simulink model "real_time_simulink_LQR"  (R2024b)
settings: Solver=ode5  StartTime=0.0  StopTime=4.5  FixedStep=0.001  RelTol=1e-3
values from neighbouring files (symbols this model uses):
  deltafil = 2^(-0.5)    (= 0.707106781187)    [LQR_code.m]    (also in PID_Luca.m)
  Klqr2 = lqr(sysG,Q,R)    [LQR_code.m]
  Nu = N(5)    [LQR_code.m]
  Nx = [N(1);N(2);N(3);N(4)]    [LQR_code.m]
  omegac = 2*pi*50    (= 314.159265359)    [LQR_code.m]    (also in PID_Luca.m)
  t0 = 0.2    [Elastic_parameters_estimation.m]    (also in LQR_code.m; PID_Luca.m)
  t1 = 0.7    [Elastic_parameters_estimation.m]    (also in LQR_code.m; PID_Luca.m)
undefined symbols (not defined in the file or in its folder): degs2rpm, DiscIntNeverNeededParam, National_Instruments, PCI, pulse2deg, rpm2rads
libraries: sldrtlib x3, simulink x3
settings Model: SimulationMode=external  ExtModeTrigDuration=1000001  Creator=galeazzolu  LastModifiedBy=galeazzolu
settings DataIOCC: ReturnWorkspaceOutputs=off
settings HardwareCC: ProdBitPerLong=64  ProdHWDeviceType=Intel->x86-64 (Linux 64)
settings RTWCC: Description=Simulink Desktop Real-Time  SystemTargetFile=sldrt.tlc  TemplateMakefile=sldrt.tmf  RTWCompilerOptimization=on
settings CodeAppCC: MaxIdLength=95
settings SimulinkDesktopRealTimeCC: TargetLibSuffix=_sldrt.a  TargetPreCompLibLocation=C:\Program Files\MATLAB\R2024b\toolbox\sldrt\lib\win64  ParMdlRefBuildCompliant=on

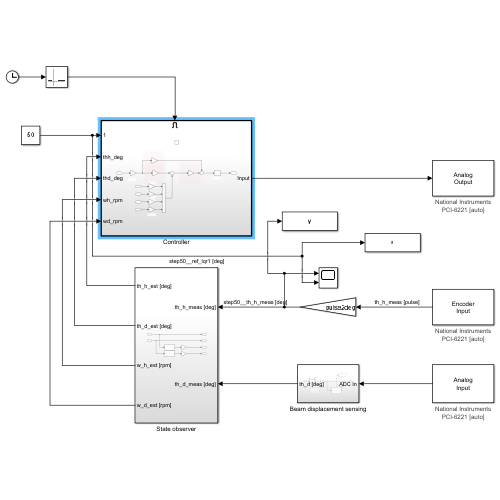
[thumbnail: Simulink's stored preview of the top-level diagram]
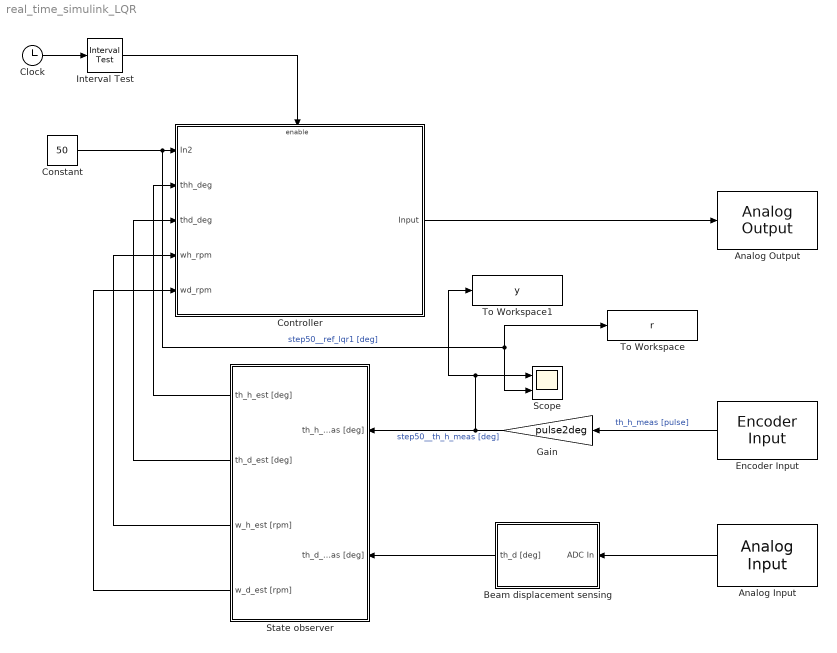
== system real_time_simulink_LQR ==
  Analog Input : sldrtlib/Analog Input  SampleTime=-1  MaxMissedTicks=10  ShowMissedTicks=off  YieldWhenWaiting=off  DrvName=National_Instruments/PCI-6221  DrvAddress=4294967295  DrvOptions=[0 0 0 2 0]  Channels=[3,4]  RangeMode=1  VoltRange=2  DataType=1
      settings: AttributesFormatString=National Instruments\nPCI-6221 [auto]
  Analog Output : sldrtlib/Analog Output  SampleTime=-1  MaxMissedTicks=10  ShowMissedTicks=off  YieldWhenWaiting=off  DrvName=National_Instruments/PCI-6221  DrvAddress=4294967295  DrvOptions=[0 0 0 2 0]  Channels=1  RangeMode=1  VoltRange=1  InitialValue=0  FinalValue=0
      settings: AttributesFormatString=National Instruments\nPCI-6221 [auto]
  Beam displacement sensing : Subsystem
  Clock : Clock
  Constant : Constant  Value=50
  Controller : Subsystem
  Encoder Input : sldrtlib/Encoder Input  SampleTime=-1  MaxMissedTicks=10  ShowMissedTicks=off  YieldWhenWaiting=off  DrvName=National_Instruments/PCI-6221  DrvAddress=4294967295  DrvOptions=[0 0 0 2 0]  Channels=1  QuadMode=3  IndexPulse=1  InputFilter=Inf  DataType=1
      settings: AttributesFormatString=National Instruments\nPCI-6221 [auto]
  Gain : Gain  Gain=pulse2deg
  Interval Test : simulink/Logic and Bit Operations/Interval Test  IntervalClosedRight=on  uplimit=inf  IntervalClosedLeft=on  lowlimit=0.7  OutDataTypeStr=boolean
  Scope : Scope  NumInputPorts=2
  State observer : Subsystem
  To Workspace : ToWorkspace  VariableName=r  SaveFormat=Structure With Time  SampleTime=-1
  To Workspace1 : ToWorkspace  VariableName=y  SaveFormat=Structure With Time  SampleTime=-1
  wires:
  Beam displacement sensing/1(th_d [deg]) -> State observer/2(th_d_meas [deg])
  Gain/1 -> To Workspace1/1, Scope/1, State observer/1(th_h_meas [deg])  "step50__th_h_meas [deg]"
  State observer/2(th_d_est [deg]) -> Controller/3(thd_deg)
  State observer/1(th_h_est [deg]) -> Controller/2(thh_deg)
  Encoder Input/1 -> Gain/1  "th_h_meas [pulse]"
  State observer/4(w_d_est [rpm]) -> Controller/5(wd_rpm)
  Analog Input/1 -> Beam displacement sensing/1(ADC In)
  State observer/3(w_h_est [rpm]) -> Controller/4(wh_rpm)
  Clock/1 -> Interval Test/1
  Interval Test/1 -> Controller/Enable
  Constant/1 -> To Workspace/1, Scope/2, Controller/1(In2)  "step50__ref_lqr1 [deg]"
  Controller/1(Input) -> Analog Output/1

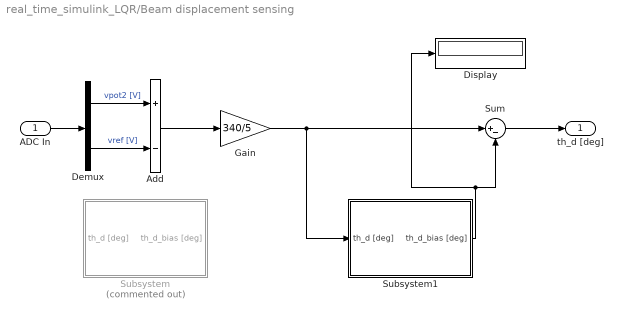
== system real_time_simulink_LQR/Beam displacement sensing ==
  ADC In : Inport
  Add : Sum  Inputs=+-
  Demux : Demux  Outputs=2
  Display : Display
  Gain : Gain  Gain=340/5
  Subsystem : Subsystem  Commented=on
  Subsystem1 : Subsystem
  Sum : Sum  Inputs=|+-
  th_d [deg] : Outport
  wires:
  ADC In/1 -> Demux/1
  Demux/1 -> Add/1  "vpot2 [V]"
  Demux/2 -> Add/2  "vref [V]"
  Add/1 -> Gain/1
  Gain/1 -> Sum/1, Subsystem1/1(th_d [deg])
  Sum/1 -> th_d [deg]/1
  Subsystem1/1(th_d_bias [deg]) -> Sum/2, Display/1

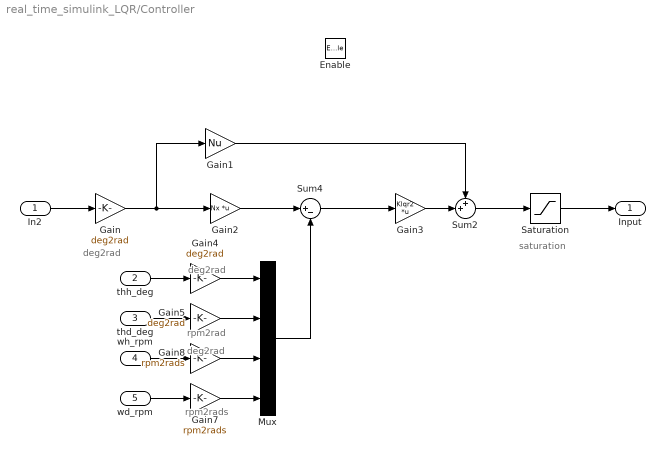
== system real_time_simulink_LQR/Controller ==
  note: rpm2rad
  note: deg2rad
  note: deg2rad
  note: deg2rad
  note: saturation
  note: rpm2rads
  In2 : Inport  PortDimensions=1
  thh_deg : Inport  Port=2
  thd_deg : Inport  Port=3
  wh_rpm : Inport  Port=4
  wd_rpm : Inport  Port=5
  Enable : EnablePort
  Gain : Gain  Gain=deg2rad
  Gain1 : Gain  Gain=Nu
  Gain2 : Gain  Gain=Nx  Multiplication=Matrix(K*u)
  Gain3 : Gain  Gain=Klqr2  Multiplication=Matrix(K*u)
  Gain4 : Gain  Gain=deg2rad
  Gain5 : Gain  Gain=deg2rad
  Gain7 : Gain  Gain=rpm2rads
  Gain8 : Gain  Gain=rpm2rads
  Mux : Mux
  Saturation : Saturate  UpperLimit=12  LowerLimit=-12  ZeroCross=off
  Sum2 : Sum  Inputs=++|
  Sum4 : Sum  Inputs=|+-
  Input : Outport  PortDimensions=1
  wires:
  thd_deg/1 -> Gain5/1
  Gain4/1 -> Mux/1
  thh_deg/1 -> Gain4/1
  Gain5/1 -> Mux/2
  Gain/1 -> Gain1/1, Gain2/1
  Saturation/1 -> Input/1
  Sum2/1 -> Saturation/1
  Gain1/1 -> Sum2/1
  Gain3/1 -> Sum2/2
  Gain2/1 -> Sum4/1
  Mux/1 -> Sum4/2
  In2/1 -> Gain/1
  Sum4/1 -> Gain3/1
  Gain7/1 -> Mux/4
  wh_rpm/1 -> Gain8/1
  Gain8/1 -> Mux/3
  wd_rpm/1 -> Gain7/1

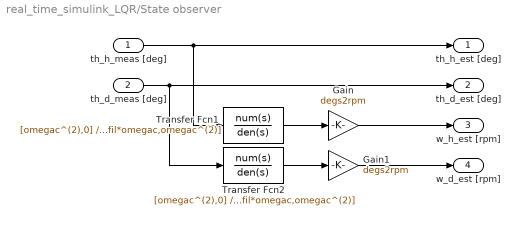
== system real_time_simulink_LQR/State observer ==
  th_h_meas [deg] : Inport
  th_d_meas [deg] : Inport  Port=2
  Gain : Gain  Gain=degs2rpm
  Gain1 : Gain  Gain=degs2rpm
  Transfer Fcn1 : TransferFcn  Numerator=[omegac^(2),0]  Denominator=[1,2*deltafil*omegac,omegac^(2)]
  Transfer Fcn2 : TransferFcn  Numerator=[omegac^(2),0]  Denominator=[1,2*deltafil*omegac,omegac^(2)]
  th_h_est [deg] : Outport
  th_d_est [deg] : Outport  Port=2
  w_h_est [rpm] : Outport  Port=3
  w_d_est [rpm] : Outport  Port=4
  wires:
  th_h_meas [deg]/1 -> Transfer Fcn1/1, th_h_est [deg]/1
  Gain/1 -> w_h_est [rpm]/1
  Transfer Fcn1/1 -> Gain/1
  th_d_meas [deg]/1 -> Transfer Fcn2/1, th_d_est [deg]/1
  Transfer Fcn2/1 -> Gain1/1
  Gain1/1 -> w_d_est [rpm]/1

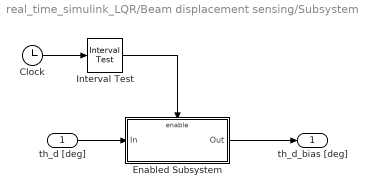
== system real_time_simulink_LQR/Beam displacement sensing/Subsystem ==
  th_d [deg] : Inport
  Clock : Clock
  Enabled Subsystem : Subsystem  TreatAsAtomicUnit=on
  Interval Test : simulink/Logic and Bit Operations/Interval Test  IntervalClosedRight=on  uplimit=t1  IntervalClosedLeft=on  lowlimit=t0  OutDataTypeStr=boolean
  th_d_bias [deg] : Outport
  wires:
  Interval Test/1 -> Enabled Subsystem/Enable
  Clock/1 -> Interval Test/1
  th_d [deg]/1 -> Enabled Subsystem/1(In)
  Enabled Subsystem/1(Out) -> th_d_bias [deg]/1

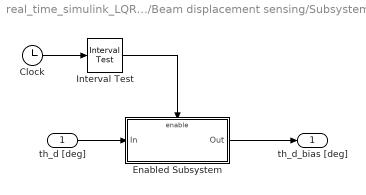
== system real_time_simulink_LQR/Beam displacement sensing/Subsystem1 ==
  th_d [deg] : Inport
  Clock : Clock
  Enabled Subsystem : Subsystem  TreatAsAtomicUnit=on
  Interval Test : simulink/Logic and Bit Operations/Interval Test  IntervalClosedRight=on  uplimit=t1  IntervalClosedLeft=on  lowlimit=t0  OutDataTypeStr=boolean
  th_d_bias [deg] : Outport
  wires:
  Enabled Subsystem/1(Out) -> th_d_bias [deg]/1
  th_d [deg]/1 -> Enabled Subsystem/1(In)
  Clock/1 -> Interval Test/1
  Interval Test/1 -> Enabled Subsystem/Enable

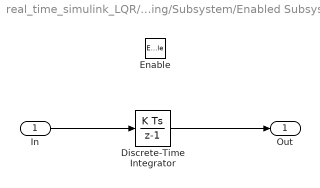
== system real_time_simulink_LQR/Beam displacement sensing/Subsystem/Enabled Subsystem ==
  In : Inport
  Enable : EnablePort
  Discrete-Time Integrator : DiscreteIntegrator  gainval=1/(t1-t0)  SampleTime=-1  ICPrevOutput=DiscIntNeverNeededParam  ICPrevScaledInput=DiscIntNeverNeededParam
  Out : Outport
  wires:
  In/1 -> Discrete-Time Integrator/1
  Discrete-Time Integrator/1 -> Out/1

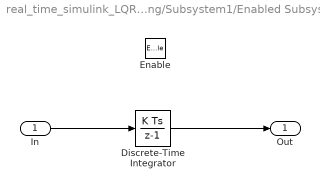
== system real_time_simulink_LQR/Beam displacement sensing/Subsystem1/Enabled Subsystem ==
  In : Inport
  Enable : EnablePort
  Discrete-Time Integrator : DiscreteIntegrator  gainval=1/(t1-t0)  SampleTime=-1  ICPrevOutput=DiscIntNeverNeededParam  ICPrevScaledInput=DiscIntNeverNeededParam
  Out : Outport
  wires:
  Discrete-Time Integrator/1 -> Out/1
  In/1 -> Discrete-Time Integrator/1
